simulink library "Generator_Lib"  (R2014a)
settings: Solver=ode45  StartTime=0.0  StopTime=10.0  RelTol=1e-3
undefined symbols (not defined in the file): block_angle, D1, Delta, DiscIntNeverNeededParam, fao, gcbh, sps_rtmsupport, Ts
libraries: powerlib x73, simulink x16, powerlib_extras x13, Generator_Lib x3, sps_avr x2, powerlib_meascontrol x2, spsSimpleSynchronousMachineModel x2
(part 2 of 3)

== system Generator_Lib/Cyclo Gen/Ideal/Phase C Cycloconverter ==
  negative cycle : powerlib/Power Electronics/Universal Bridge  Arms=3  SnubberResistance=1e3  SnubberCapacitance=1e-7  Device=Thyristors  Ron=1e-5  Lon=0  ForwardVoltages="[  0  0  ]"  ForwardVoltage=0  GTOparameters=[ 10e-6 , 20e-6 ]  IGBTparameters=[ 1e-6 , 2e-6 ]  Measurements=None  Measurements_2=None  converterType=Rectifier
  positive cycle : powerlib/Power Electronics/Universal Bridge  Arms=3  SnubberResistance=1e3  SnubberCapacitance=1e-7  Device=Thyristors  Ron=1e-5  Lon=0  ForwardVoltages="[  0  0  ]"  ForwardVoltage=0  GTOparameters=[ 10e-6 , 20e-6 ]  IGBTparameters=[ 1e-6 , 2e-6 ]  Measurements=None  Measurements_2=None  converterType=Rectifier
  VC+ : PMIOPort  Tag=PMCPort  Port=1  Side=Right
  VC- : PMIOPort  Tag=PMCPort  Port=2  Side=Right
  A : PMIOPort  Tag=PMCPort  Port=3  Side=Left
  B : PMIOPort  Tag=PMCPort  Port=4  Side=Left
  C : PMIOPort  Tag=PMCPort  Port=5  Side=Left
  wires:
  [PhCgp] -> positive cycle/1
  [PhCgn] -> negative cycle/1
  connections:
  A/RConn1 -- positive cycle/LConn1 -- negative cycle/LConn1
  B/RConn1 -- positive cycle/LConn2 -- negative cycle/LConn2
  C/RConn1 -- positive cycle/LConn3 -- negative cycle/LConn3
  negative cycle/RConn1 -- positive cycle/RConn2 -- VC-/RConn1
  positive cycle/RConn1 -- VC+/RConn1 -- negative cycle/RConn2

== system Generator_Lib/DC Gen/Ideal/Sensing ==
  Constant : Constant  Value=[1 1]*12000  SampleTime=-1
  Constant1 : Constant  Value=202  SampleTime=-1
  Mux : Mux  Inputs=3
  rpm2pu1 : Gain  Gain=2*pi/60
  tag scope: Gen1Data=global
  wires:
  Constant/1 -> rpm2pu1/1  "Spd"
  Mux/1 -> [Gen1Data]
  rpm2pu1/1 -> Mux/1
  Constant1/1 -> Mux/2
  [Pwr_Gen1_Only] -> Mux/3

== system Generator_Lib/DC Gen/Sync Mach/Displays ==
  w : Inport
  Frequency (Hz) : Display
      settings: Decimation=100  SampleTime=1e-2
  Gain : Gain  Gain=30/pi
  Gain3 : Gain  Gain=1/30
  Rate Transition : RateTransition  OutPortSampleTimeOpt=Inherit  OutPortSampleTime=Ts
  Rate Transition1 : RateTransition  OutPortSampleTimeOpt=Inherit  OutPortSampleTime=Ts
  Speed (RPM) : Display
      settings: Decimation=100  SampleTime=1e-2
  wires:
  w/1 -> Gain/1
  Rate Transition/1 -> Speed (RPM)/1
  Gain3/1 -> Rate Transition1/1
  Gain/1 -> Rate Transition/1, Gain3/1
  Rate Transition1/1 -> Frequency (Hz)/1

== system Generator_Lib/DC Gen/Sync Mach/Generator Control Unit (GCU) ==
  Iabc : Inport
  Vabc : Inport  Port=2
  PMG : Inport  Port=3
  Demux : Demux  Outputs=3
  Excitation System : sps_avr/Excitation System  tr=20e-3  reg=[ 300, 0.001 ]  exc=[ 1, 0 ]  tgr=[ 0, 0 ]  damp=[ 0.001, 0.1 ]  sat=[ 0, 0 ]  lim=[ -2, 2, 0 ]  v0=[1 1*203.1/200]
  Integrator : Integrator
  PU_SI : Gain  Gain=200
  SI_PU : Gain  Gain=1/(200*sqrt(2))
  Terminator1 : Terminator
  Terminator2 : Terminator
  Vref : Constant
  abc to dq0 : powerlib_meascontrol/Transformations/abc to dq0  Alignment=90 degrees behind phase A axis
  threshold3 : Constant  Value=0
  V Field : Outport
  tag scope: Gen1_Vfield=global
  wires:
  Vabc/1 -> SI_PU/1
  PMG/1 -> Integrator/1
  Integrator/1 -> abc to dq0/2
  abc to dq0/1 -> Demux/1
  Demux/1 -> Excitation System/2
  Demux/2 -> Excitation System/3
  SI_PU/1 -> abc to dq0/1
  Excitation System/1 -> PU_SI/1
  PU_SI/1 -> V Field/1, [Gen1_Vfield]
  Vref/1 -> Excitation System/1
  threshold3/1 -> Excitation System/4
  Iabc/1 -> Terminator1/1
  Demux/3 -> Terminator2/1

== system Generator_Lib/DC Gen/Sync Mach/Generator Control Breaker (GCB) ==
  GLC : Inport
  Close switch : Subsystem
  Complex to Real-Imag : ComplexToRealImag  Output=Real
  Complex to Real-Imag1 : ComplexToRealImag  Output=Real
  Contactor : Subsystem
  Memory : Memory
  P.O.R  and CTA : powerlib/Measurements/Three-Phase V-I Measurement  VoltageMeasurement=phase-to-phase  SetLabelV=off  LabelV=Vabc_Gen1  Vpu=off  VpuLL=off  CurrentMeasurement=yes  SetLabelI=off  LabelI=Iabc_Gen1  Ipu=off  Pbase=100e6  Vbase=500e3  OutputType=Complex  PhasorSimulation=off  PSBequivalent=0
  in_a : PMIOPort  Port=1  Side=Left
  in_b : PMIOPort  Port=2  Side=Left
  in_c : PMIOPort  Port=3  Side=Left
  out_a : PMIOPort  Port=4  Side=Right
  out_b : PMIOPort  Port=5  Side=Right
  out_c : PMIOPort  Port=6  Side=Right
  Vabc : Outport
  Iabc : Outport  Port=2
  wires:
  Close switch/1(Out1) -> Contactor/1(com)
  Memory/1 -> Close switch/1(In1)
  Complex to Real-Imag1/1 -> Iabc/1
  Complex to Real-Imag/1 -> Vabc/1
  P.O.R  and CTA/2 -> Complex to Real-Imag1/1
  P.O.R  and CTA/1 -> Complex to Real-Imag/1
  GLC/1 -> Memory/1
  connections:
  Contactor/RConn3 -- out_c/RConn1
  Contactor/RConn1 -- out_a/RConn1
  P.O.R  and CTA/RConn2 -- Contactor/LConn2
  Contactor/LConn3 -- P.O.R  and CTA/RConn3
  P.O.R  and CTA/LConn3 -- in_c/RConn1
  in_b/RConn1 -- P.O.R  and CTA/LConn2
  P.O.R  and CTA/LConn1 -- in_a/RConn1
  Contactor/LConn1 -- P.O.R  and CTA/RConn1
  out_b/RConn1 -- Contactor/RConn2

== system Generator_Lib/DC Gen/Sync Mach/Sensing ==
  In1 : Inport
  Data : Subsystem
  Mux : Mux  Inputs=3
  tag scope: Gen1Data=global
  wires:
  Mux/1 -> [Gen1Data]
  In1/1 -> Data/1(B)
  Data/1(w) -> Mux/1
  Data/2(Vf) -> Mux/2
  Data/3(Pe) -> Mux/3

== system Generator_Lib/DC Gen/Sync Mach/Simplified Synchronous Machine SI Units ==
  mec : Inport
  E : Inport  Port=2
  Electrical model : Subsystem  BlockChoice=Continuous
      settings: AttributesFormatString=%<BlockChoice>  TemplateBlock=spsSimpleSynchronousMachineModel/Electrical model  MemberBlocks=Continuous,Discrete,Phasor
  Measurement list : Subsystem
  Mechanical model : Subsystem  BlockChoice=Continuous w input
      settings: AttributesFormatString=%<BlockChoice>  TemplateBlock=spsSimpleSynchronousMachineModel/Mechanical model  MemberBlocks=Continuous Pm input,Continuous w input,Discrete Pm input,Discrete w input,Phasor Pm input,Phasor w input,Shaft input
  SSM : PMComponent  PhysicalDomain=powersysdomain  LeftPortType=p1  RightPortType=p1  LConnTagsString=__newl0  RConnTagsString=A|B|C  mask(InnerPowersysBlock){}
  A : PMIOPort  Port=1  Side=Right
  B : PMIOPort  Port=2  Side=Right
  C : PMIOPort  Port=3  Side=Right
  m : Outport  InitialOutput=0
  tag scope: LibraryTag=global
  wires:
  Mechanical model/2(wm) -> Electrical model/4(wm)
  Mechanical model/1(theta_e) -> Electrical model/3(theta_e)
  E/1 -> Electrical model/2(e)
  [LibraryTag] -> Electrical model/1(v)
  Electrical model/1(i) -> [LibraryTag]
  Electrical model/2(m) -> Measurement list/1(In1)
  mec/1 -> Mechanical model/1(input)  "Pm or w"
  Electrical model/3(Pe) -> Mechanical model/2(Pe)
  Measurement list/1(Out1) -> m/1
  connections:
  SSM/RConn2 -- B/RConn1
  SSM/RConn1 -- A/RConn1
  SSM/RConn3 -- C/RConn1

== system Generator_Lib/DC Gen/Sync Mach/Vab ==
  Voltage Measurement : powerlib/Measurements/Voltage Measurement  PhasorSimulation=off  OutputType=Magnitude  PSBequivalent=0
  + : PMIOPort  Port=1  Side=Right
  - : PMIOPort  Port=2  Side=Right
  tag scope: Gen1_Vab=global
  wires:
  Voltage Measurement/1 -> [Gen1_Vab]
  connections:
  Voltage Measurement/LConn2 -- -/RConn1
  Voltage Measurement/LConn1 -- +/RConn1

== system Generator_Lib/Integrated Drive/Generator Control Breaker (GCB)/Close switch ==
  In1 : Inport
  Data Type Conversion : DataTypeConversion
  Rad_Rpm : Gain  Gain=30/pi
  Relay : Relay  OnSwitchValue=9000  OffSwitchValue=8900
  Out1 : Outport
  wires:
  In1/1 -> Rad_Rpm/1
  Relay/1 -> Data Type Conversion/1
  Rad_Rpm/1 -> Relay/1
  Data Type Conversion/1 -> Out1/1

== system Generator_Lib/Integrated Drive/Generator Control Breaker (GCB)/Contactor ==
  com : Inport
  Three-Phase Breaker : powerlib/Elements/Three-Phase Breaker  InitialState=open  SwitchA=on  SwitchB=on  SwitchC=on  SwitchTimes="[4/60  10/60]"  External=on  BreakerResistance=0.001  SnubberResistance=1e3  SnubberCapacitance=inf  Measurements=None
  A : PMIOPort  Port=1  Side=Left
  a : PMIOPort  Port=2  Side=Right
  B : PMIOPort  Port=3  Side=Left
  b : PMIOPort  Port=4  Side=Right
  C : PMIOPort  Port=5  Side=Left
  c : PMIOPort  Port=6  Side=Right
  wires:
  com/1 -> Three-Phase Breaker/1
  connections:
  C/RConn1 -- Three-Phase Breaker/LConn3
  B/RConn1 -- Three-Phase Breaker/LConn2
  A/RConn1 -- Three-Phase Breaker/LConn1
  c/RConn1 -- Three-Phase Breaker/RConn3
  Three-Phase Breaker/RConn2 -- b/RConn1
  a/RConn1 -- Three-Phase Breaker/RConn1

== system Generator_Lib/Integrated Drive/Sensing/Data ==
  B : Inport
  Bus Selector : BusSelector  OutputSignals=Rotor speed wm (rad/s),Electrical power Pe (W),Terminal voltage Va (V),Terminal voltage Vb (V),Terminal voltage Vc (V),Stator current is_a (A),Stator current is_b (A),Stator current is_c (A)
  Constant : Constant  Value=12000
  Mux : Mux  Inputs=2
  Mux1 : Mux  Inputs=3
  Mux2 : Mux  Inputs=3
  rpm2pu1 : Gain  Gain=2*pi/60
  w : Outport
  Vf : Outport  Port=2
  Pe : Outport  Port=3
  tag scope: Iabc_Gen1Only=global, Vabc_Gen1Only=global
  wires:
  [Gen1_Vfield] -> Vf/1
  B/1 -> Bus Selector/1
  Bus Selector/2 -> Pe/1  "<Electrical power Pe (W)>"
  Bus Selector/1 -> Mux/1  "<Rotor speed wm (rad/s)>"
  rpm2pu1/1 -> Mux/2
  Constant/1 -> rpm2pu1/1  "Spd"
  Mux/1 -> w/1
  Bus Selector/3 -> Mux1/1  "<Terminal voltage Va (V)>"
  Bus Selector/4 -> Mux1/2  "<Terminal voltage Vb (V)>"
  Bus Selector/5 -> Mux1/3  "<Terminal voltage Vc (V)>"
  Mux1/1 -> [Vabc_Gen1Only]
  Mux2/1 -> [Iabc_Gen1Only]
  Bus Selector/6 -> Mux2/1  "<Stator current is_a (A)>"
  Bus Selector/7 -> Mux2/2  "<Stator current is_b (A)>"
  Bus Selector/8 -> Mux2/3  "<Stator current is_c (A)>"

== system Generator_Lib/VSCF Cycloconverter/AC Generator Cycloconverter/Cycloconverter control (Vsync) ==
  Cyclo Firing Control PhA : Subsystem
  Cyclo Firing Control PhB : Subsystem
  Cyclo Firing Control PhC : Subsystem
  Demux : Demux  Outputs=3
  Discrete-Time Integrator : DiscreteIntegrator  SampleTime=Ts  ICPrevOutput=DiscIntNeverNeededParam  ICPrevScaledInput=DiscIntNeverNeededParam
  Gain1 : Gain  Gain=2*pi
  Gain2 : Gain  Gain=1/(200*sqrt(2/3))
  Gain5 : Gain  Gain=200*sqrt(2/3)
  Sine : Subsystem
  output frequency (Hz) : simulink/Sources/Repeating Sequence  rep_seq_t=[0 10]  rep_seq_y=[1 1]*400
  output voltage (V peak) : simulink/Sources/Repeating Sequence  rep_seq_t=[0 10]  rep_seq_y=[1 1]*200*sqrt(2/3)
  tag scope: Ea=global, vab=global, vbc=global, vca=global
  wires:
  Discrete-Time Integrator/1 -> Sine/2(theta)
  Sine/2(b) -> Cyclo Firing Control PhB/1(Eref)
  Sine/1(a) -> Cyclo Firing Control PhA/1(Eref), Gain5/1
  Sine/3(c) -> Cyclo Firing Control PhC/1(Eref)
  output frequency (Hz)/1 -> Gain1/1
  Gain1/1 -> Discrete-Time Integrator/1
  Gain5/1 -> [Ea]
  output voltage (V peak)/1 -> Gain2/1
  Gain2/1 -> Sine/1(Eref)
  [Vsync] -> Demux/1
  Demux/1 -> [vab]
  Demux/2 -> [vbc]
  Demux/3 -> [vca]
  [input_freq] -> Cyclo Firing Control PhC/2(freq (Hz)), Cyclo Firing Control PhA/2(freq (Hz)), Cyclo Firing Control PhB/2(freq (Hz))

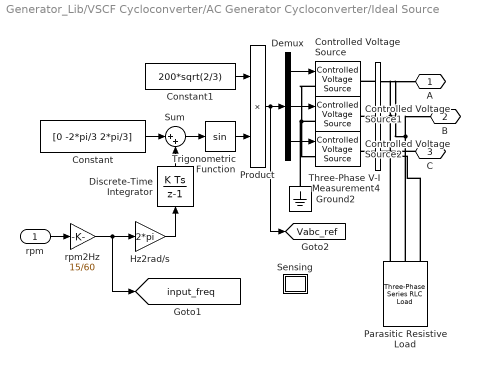
== system Generator_Lib/VSCF Cycloconverter/AC Generator Cycloconverter/Ideal Source ==
  rpm : Inport
  Constant : Constant  Value=[0 -2*pi/3 2*pi/3]
  Constant1 : Constant  Value=200*sqrt(2/3)
  Controlled Voltage Source : powerlib/Electrical Sources/Controlled Voltage Source  Initialize=off  Source_Type=AC  Amplitude=0  Phase=0  Frequency=0  Measurements=None
  Controlled Voltage Source1 : powerlib/Electrical Sources/Controlled Voltage Source  Initialize=off  Source_Type=AC  Amplitude=0  Phase=0  Frequency=0  Measurements=None
  Controlled Voltage Source2 : powerlib/Electrical Sources/Controlled Voltage Source  Initialize=off  Source_Type=AC  Amplitude=0  Phase=0  Frequency=0  Measurements=None
  Demux : Demux  Outputs=3
  Discrete-Time Integrator : DiscreteIntegrator  SampleTime=Ts  ICPrevOutput=DiscIntNeverNeededParam  ICPrevScaledInput=DiscIntNeverNeededParam
  Ground2 : powerlib/Elements/Ground  LConnTagsString=a
  Hz2rad/s : Gain  Gain=2*pi
  Parasitic Resistive Load : powerlib/Elements/Three-Phase Series RLC Load  LConnTagsString=A|B|C  Configuration=Y (grounded)  NominalVoltage=200  NominalFrequency=400  ActivePower=5000  InductivePower=0  CapacitivePower=0  Measurements=None  LoadType=constant Z
  Product : Product
  Sensing : Subsystem
      mask Display: disp('S')
  Sum : Sum  Inputs=|++
  Three-Phase V-I Measurement4 : powerlib/Measurements/Three-Phase V-I Measurement  VoltageMeasurement=phase-to-ground  SetLabelV=on  LabelV=Vabc_Gen1Only  Vpu=off  VpuLL=off  CurrentMeasurement=yes  SetLabelI=on  LabelI=Iabc_Gen1Only  Ipu=off  Pbase=100e6  Vbase=500e3  OutputType=Magnitude  PhasorSimulation=on  PSBequivalent=0
  Trigonometric Function : Trigonometry
  rpm2Hz : Gain  Gain=15/60
  A : PMIOPort  Port=1  Side=Right
  B : PMIOPort  Port=2  Side=Right
  C : PMIOPort  Port=3  Side=Right
  tag scope: Vabc_ref=global, input_freq=global
  wires:
  rpm/1 -> rpm2Hz/1
  Discrete-Time Integrator/1 -> Sum/2
  Constant1/1 -> Product/1
  Constant/1 -> Sum/1
  Hz2rad/s/1 -> Discrete-Time Integrator/1
  Sum/1 -> Trigonometric Function/1
  Trigonometric Function/1 -> Product/2
  Product/1 -> [Vabc_ref], Demux/1
  Demux/1 -> Controlled Voltage Source/1
  Demux/2 -> Controlled Voltage Source1/1
  Demux/3 -> Controlled Voltage Source2/1
  rpm2Hz/1 -> [input_freq], Hz2rad/s/1
  connections:
  Controlled Voltage Source/LConn1 -- Ground2/LConn1 -- Controlled Voltage Source2/LConn1 -- Controlled Voltage Source1/LConn1
  Three-Phase V-I Measurement4/LConn2 -- Controlled Voltage Source1/RConn1
  Three-Phase V-I Measurement4/LConn1 -- Controlled Voltage Source/RConn1
  Three-Phase V-I Measurement4/LConn3 -- Controlled Voltage Source2/RConn1
  C/RConn1 -- Parasitic Resistive Load/LConn3 -- Three-Phase V-I Measurement4/RConn3
  Three-Phase V-I Measurement4/RConn2 -- B/RConn1 -- Parasitic Resistive Load/LConn2
  Three-Phase V-I Measurement4/RConn1 -- A/RConn1 -- Parasitic Resistive Load/LConn1

== system Generator_Lib/VSCF Cycloconverter/AC Generator Cycloconverter/Phase A Cycloconverter ==
  negative cycle : powerlib/Power Electronics/Universal Bridge  Arms=3  SnubberResistance=1e3  SnubberCapacitance=1e-7  Device=Thyristors  Ron=1e-5  Lon=0  ForwardVoltages="[  0  0  ]"  ForwardVoltage=0  GTOparameters=[ 10e-6 , 20e-6 ]  IGBTparameters=[ 1e-6 , 2e-6 ]  Measurements=None  Measurements_2=None  converterType=Rectifier
  positive cycle : powerlib/Power Electronics/Universal Bridge  Arms=3  SnubberResistance=1e3  SnubberCapacitance=1e-7  Device=Thyristors  Ron=1e-5  Lon=0  ForwardVoltages="[  0  0  ]"  ForwardVoltage=0  GTOparameters=[ 10e-6 , 20e-6 ]  IGBTparameters=[ 1e-6 , 2e-6 ]  Measurements=None  Measurements_2=None  converterType=Rectifier
  VA+ : PMIOPort  Tag=PMCPort  Port=1  Side=Right
  VA- : PMIOPort  Tag=PMCPort  Port=2  Side=Right
  A : PMIOPort  Tag=PMCPort  Port=3  Side=Left
  B : PMIOPort  Tag=PMCPort  Port=4  Side=Left
  C : PMIOPort  Tag=PMCPort  Port=5  Side=Left
  wires:
  [PhAgp] -> positive cycle/1
  [PhAgn] -> negative cycle/1
  connections:
  A/RConn1 -- positive cycle/LConn1 -- negative cycle/LConn1
  B/RConn1 -- positive cycle/LConn2 -- negative cycle/LConn2
  C/RConn1 -- positive cycle/LConn3 -- negative cycle/LConn3
  negative cycle/RConn1 -- positive cycle/RConn2 -- VA-/RConn1
  positive cycle/RConn1 -- VA+/RConn1 -- negative cycle/RConn2

== system Generator_Lib/VSCF Cycloconverter/AC Generator Cycloconverter/Phase B Cycloconverter ==
  negative cycle : powerlib/Power Electronics/Universal Bridge  Arms=3  SnubberResistance=1e3  SnubberCapacitance=1e-7  Device=Thyristors  Ron=1e-5  Lon=0  ForwardVoltages="[  0  0  ]"  ForwardVoltage=0  GTOparameters=[ 10e-6 , 20e-6 ]  IGBTparameters=[ 1e-6 , 2e-6 ]  Measurements=None  Measurements_2=None  converterType=Rectifier
  positive cycle : powerlib/Power Electronics/Universal Bridge  Arms=3  SnubberResistance=1e3  SnubberCapacitance=1e-7  Device=Thyristors  Ron=1e-5  Lon=0  ForwardVoltages="[  0  0  ]"  ForwardVoltage=0  GTOparameters=[ 10e-6 , 20e-6 ]  IGBTparameters=[ 1e-6 , 2e-6 ]  Measurements=None  Measurements_2=None  converterType=Rectifier
  VB+ : PMIOPort  Tag=PMCPort  Port=1  Side=Right
  VB- : PMIOPort  Tag=PMCPort  Port=2  Side=Right
  A : PMIOPort  Tag=PMCPort  Port=3  Side=Left
  B : PMIOPort  Tag=PMCPort  Port=4  Side=Left
  C : PMIOPort  Tag=PMCPort  Port=5  Side=Left
  wires:
  [PhBgn] -> negative cycle/1
  [PhBgp] -> positive cycle/1
  connections:
  negative cycle/RConn2 -- VB+/RConn1 -- positive cycle/RConn1
  VB-/RConn1 -- positive cycle/RConn2 -- negative cycle/RConn1
  negative cycle/LConn3 -- positive cycle/LConn3 -- C/RConn1
  negative cycle/LConn2 -- B/RConn1 -- positive cycle/LConn2
  negative cycle/LConn1 -- positive cycle/LConn1 -- A/RConn1

== system Generator_Lib/VSCF Cycloconverter/AC Generator Cycloconverter/Phase C Cycloconverter ==
  negative cycle : powerlib/Power Electronics/Universal Bridge  Arms=3  SnubberResistance=1e3  SnubberCapacitance=1e-7  Device=Thyristors  Ron=1e-5  Lon=0  ForwardVoltages="[  0  0  ]"  ForwardVoltage=0  GTOparameters=[ 10e-6 , 20e-6 ]  IGBTparameters=[ 1e-6 , 2e-6 ]  Measurements=None  Measurements_2=None  converterType=Rectifier
  positive cycle : powerlib/Power Electronics/Universal Bridge  Arms=3  SnubberResistance=1e3  SnubberCapacitance=1e-7  Device=Thyristors  Ron=1e-5  Lon=0  ForwardVoltages="[  0  0  ]"  ForwardVoltage=0  GTOparameters=[ 10e-6 , 20e-6 ]  IGBTparameters=[ 1e-6 , 2e-6 ]  Measurements=None  Measurements_2=None  converterType=Rectifier
  VC+ : PMIOPort  Tag=PMCPort  Port=1  Side=Right
  VC- : PMIOPort  Tag=PMCPort  Port=2  Side=Right
  A : PMIOPort  Tag=PMCPort  Port=3  Side=Left
  B : PMIOPort  Tag=PMCPort  Port=4  Side=Left
  C : PMIOPort  Tag=PMCPort  Port=5  Side=Left
  wires:
  [PhCgp] -> positive cycle/1
  [PhCgn] -> negative cycle/1
  connections:
  A/RConn1 -- positive cycle/LConn1 -- negative cycle/LConn1
  B/RConn1 -- positive cycle/LConn2 -- negative cycle/LConn2
  C/RConn1 -- positive cycle/LConn3 -- negative cycle/LConn3
  negative cycle/RConn1 -- positive cycle/RConn2 -- VC-/RConn1
  positive cycle/RConn1 -- VC+/RConn1 -- negative cycle/RConn2

== system Generator_Lib/VSCF Cycloconverter/Generator Control Breaker (GCB)/Close switch ==
  In1 : Inport
  Data Type Conversion : DataTypeConversion
  Rad_Rpm : Gain  Gain=30/pi
  Relay : Relay  OnSwitchValue=9000  OffSwitchValue=8900
  Out1 : Outport
  wires:
  In1/1 -> Rad_Rpm/1
  Relay/1 -> Data Type Conversion/1
  Rad_Rpm/1 -> Relay/1
  Data Type Conversion/1 -> Out1/1

== system Generator_Lib/VSCF Cycloconverter/Generator Control Breaker (GCB)/Contactor ==
  com : Inport
  Three-Phase Breaker : powerlib/Elements/Three-Phase Breaker  InitialState=open  SwitchA=on  SwitchB=on  SwitchC=on  SwitchTimes="[4/60  10/60]"  External=on  BreakerResistance=0.001  SnubberResistance=1e3  SnubberCapacitance=inf  Measurements=None
  A : PMIOPort  Port=1  Side=Left
  a : PMIOPort  Port=2  Side=Right
  B : PMIOPort  Port=3  Side=Left
  b : PMIOPort  Port=4  Side=Right
  C : PMIOPort  Port=5  Side=Left
  c : PMIOPort  Port=6  Side=Right
  wires:
  com/1 -> Three-Phase Breaker/1
  connections:
  C/RConn1 -- Three-Phase Breaker/LConn3
  B/RConn1 -- Three-Phase Breaker/LConn2
  A/RConn1 -- Three-Phase Breaker/LConn1
  c/RConn1 -- Three-Phase Breaker/RConn3
  Three-Phase Breaker/RConn2 -- b/RConn1
  a/RConn1 -- Three-Phase Breaker/RConn1

== system Generator_Lib/VSCF DC Link/Rect and Inv/Subsystem3 ==
  Vdc : powerlib/Measurements/Voltage Measurement  Tag=PoWeRsYsTeMmEaSuReMeNt  PhasorSimulation=off  OutputType=Magnitude  PSBequivalent=0
  + : PMIOPort  Port=1  Side=Left
  - : PMIOPort  Port=2  Side=Right
  tag scope: Vdc_GenDCLink=global
  wires:
  Vdc/1 -> [Vdc_GenDCLink]  "Vdc"
  connections:
  Vdc/LConn1 -- +/RConn1
  -/RConn1 -- Vdc/LConn2

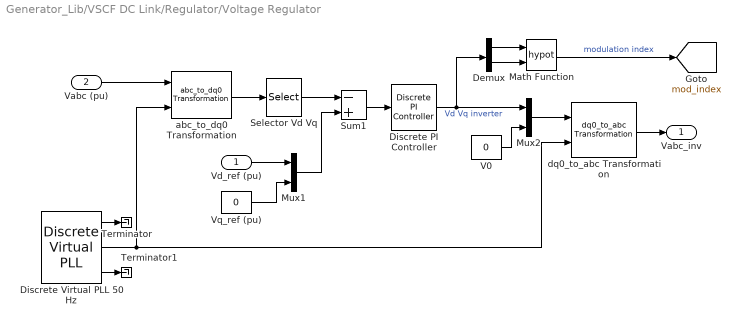
== system Generator_Lib/VSCF DC Link/Regulator/Voltage Regulator ==
  Vd_ref (pu) : Inport
  Vabc (pu) : Inport  Port=2
  Demux : Demux  Outputs=2
  Discrete PI Controller : powerlib_extras/Discrete  Control Blocks/Discrete PI Controller  Kp=Kp  Ki=Ki  Par_Limits=[1 -1]  Init=0  Ts=Ts
  Discrete Virtual PLL 50 Hz : powerlib_extras/Discrete  Control Blocks/Discrete Virtual PLL  Freq=400  Phase=0  Ts=Ts
  Math Function : Math  Operator=hypot  SaturateOnIntegerOverflow=on
  Mux1 : Mux  Inputs=2
  Mux2 : Mux  Inputs=2
  Selector Vd Vq : Selector  InputPortWidth=3  Indices=[1 2]
  Sum1 : Sum  Inputs=-+  SaturateOnIntegerOverflow=on  InputSameDT=on  OutDataTypeStr=Inherit: Same as first input
  Terminator : Terminator
  Terminator1 : Terminator
  V0 : Constant  Value=0
  Vq_ref (pu) : Constant  Value=0
  abc_to_dq0 Transformation : powerlib_extras/Measurements/abc_to_dq0 Transformation
  dq0_to_abc Transformation : powerlib_extras/Measurements/dq0_to_abc Transformation
  Vabc_inv : Outport
  tag scope: mod_index=global
  wires:
  abc_to_dq0 Transformation/1 -> Selector Vd Vq/1
  Vabc (pu)/1 -> abc_to_dq0 Transformation/1
  Selector Vd Vq/1 -> Sum1/1
  Sum1/1 -> Discrete PI Controller/1
  Mux2/1 -> dq0_to_abc Transformation/1
  V0/1 -> Mux2/2
  dq0_to_abc Transformation/1 -> Vabc_inv/1
  Discrete Virtual PLL 50 Hz/2 -> abc_to_dq0 Transformation/2, dq0_to_abc Transformation/2
  Vd_ref (pu)/1 -> Mux1/1
  Vq_ref (pu)/1 -> Mux1/2
  Mux1/1 -> Sum1/2
  Discrete Virtual PLL 50 Hz/1 -> Terminator/1
  Discrete Virtual PLL 50 Hz/3 -> Terminator1/1
  Discrete PI Controller/1 -> Demux/1, Mux2/1  "Vd Vq inverter"
  Demux/1 -> Math Function/1
  Demux/2 -> Math Function/2
  Math Function/1 -> [mod_index]  "modulation index"

== system Generator_Lib/Cyclo Gen/Ideal/Cycloconverter control (Vsync)/Cyclo Firing Control PhA ==
  Eref : Inport
  freq (Hz) : Inport  Port=2
  Compare To Constant : simulink/Logic and Bit Operations/Compare To Constant  relop=>=  const=block_angle  OutDataTypeStr=boolean  ZeroCross=off
  Compare To Constant1 : simulink/Logic and Bit Operations/Compare To Constant  relop=>  const=block_angle  OutDataTypeStr=boolean  ZeroCross=off
  Discrete Synchronized 6-Pulse Generator (negative) : powerlib_extras/Discrete  Control Blocks/Discrete Synchronized 6-Pulse Generator  pwidth=150  Double_Pulse=off  Ts=Ts
  Discrete Synchronized 6-Pulse Generator (positive) : powerlib_extras/Discrete  Control Blocks/Discrete Synchronized 6-Pulse Generator  pwidth=150  Double_Pulse=off  Ts=Ts
  Gain2 : Gain  Gain=-1
  Lookup Table (negative) : Lookup  InputValues=[-1 0 1]  Table=[90 90 0]+fao
  Lookup Table (positive) : Lookup  InputValues=[-1 0 1]  Table=[90 90 0]+fao
  tag scope: PhAgn=global, PhAgp=global
  wires:
  Discrete Synchronized 6-Pulse Generator (positive)/1 -> [PhAgp]
  Discrete Synchronized 6-Pulse Generator (negative)/1 -> [PhAgn]
  [vca] -> Discrete Synchronized 6-Pulse Generator (positive)/4
  [vbc] -> Discrete Synchronized 6-Pulse Generator (positive)/3
  [vab] -> Discrete Synchronized 6-Pulse Generator (positive)/2
  [vab] -> Discrete Synchronized 6-Pulse Generator (negative)/2
  [vbc] -> Discrete Synchronized 6-Pulse Generator (negative)/3
  [vca] -> Discrete Synchronized 6-Pulse Generator (negative)/4
  Compare To Constant/1 -> Discrete Synchronized 6-Pulse Generator (positive)/6
  Lookup Table (positive)/1 -> Compare To Constant/1, Discrete Synchronized 6-Pulse Generator (positive)/1  "alpha_pos"
  Lookup Table (negative)/1 -> Discrete Synchronized 6-Pulse Generator (negative)/1, Compare To Constant1/1  "alpa_neg"
  Eref/1 -> Lookup Table (positive)/1, Gain2/1
  Compare To Constant1/1 -> Discrete Synchronized 6-Pulse Generator (negative)/6
  Gain2/1 -> Lookup Table (negative)/1
  freq (Hz)/1 -> Discrete Synchronized 6-Pulse Generator (positive)/5, Discrete Synchronized 6-Pulse Generator (negative)/5

== system Generator_Lib/Cyclo Gen/Ideal/Cycloconverter control (Vsync)/Cyclo Firing Control PhB ==
  Eref : Inport
  freq (Hz) : Inport  Port=2
  Compare To Constant : simulink/Logic and Bit Operations/Compare To Constant  relop=>=  const=block_angle  OutDataTypeStr=boolean  ZeroCross=off
  Compare To Constant1 : simulink/Logic and Bit Operations/Compare To Constant  relop=>  const=block_angle  OutDataTypeStr=boolean  ZeroCross=off
  Discrete Synchronized 6-Pulse Generator : powerlib_extras/Discrete  Control Blocks/Discrete Synchronized 6-Pulse Generator  pwidth=150  Double_Pulse=off  Ts=Ts
  Discrete Synchronized 6-Pulse Generator1 : Subsystem  DialogController=POWERSYS.PowerSysDialog  mask(Discrete Synchronized 6-pulse generator){pwidth=150, Double_Pulse=off, Ts=Ts}
      mask prompts: pwidth "Pulse width (degrees) :"; Double_Pulse "Double pulsing"; Ts "Time step (s) :"
      mask help:
      | Use this block to fire the 6 thyristors of a 6-pulse converter.
      |
      | The output is a vector of 6 pulses (0-1) individually synchronized on the 6 commutation voltages. Pulses are generated alpha degrees after the increasing zero-crossings of the commutation voltages.
      |
      | Input 1 is  the alpha firing signal (degrees).
      | Inputs 2, 3 and 4 are the synchronization voltages AB BC CA which should be in phase with the 3 phase-phase voltages at the converter terminals.
      | Input 5: Frequency of the synchronization voltages (use a constant or the Freq PLL output)
      | Input 6 allows  blocking of the pulses when the applied signal is non zero.
      |
      | When the 'Douple pulsing' option is checked, two pulses are sent to each thyristor: a 1st pulse when the aplha angle is reached, then a 2nd pulse 60 degrees later, when the next thyristor is fired.
      mask init:
      | power_initmask();
      mask Help: This block is part of a subset of blocks in the Extras library that does not have documentation associated with it, other than the block mask description.
      mask Display: plot(0,0,100,100,[80 62 62 47 47 30],[40 40 60 60 40 40]-5)
  Gain2 : Gain  Gain=-1
  Lookup Table : Lookup  InputValues=[-1 0 1]  Table=[90 90 0]+fao
  Lookup Table1 : Lookup  InputValues=[-1 0 1]  Table=[90 90 0]+fao
  tag scope: PhBgn=global, PhBgp=global
  wires:
  Eref/1 -> Lookup Table/1, Gain2/1
  Lookup Table1/1 -> Compare To Constant1/1, Discrete Synchronized 6-Pulse Generator1/1(alpha_deg)  "alpa_neg_B"
  Lookup Table/1 -> Compare To Constant/1, Discrete Synchronized 6-Pulse Generator/1  "alpha_pos_B"
  Compare To Constant/1 -> Discrete Synchronized 6-Pulse Generator/6
  [vca] -> Discrete Synchronized 6-Pulse Generator1/4(CA)
  [vbc] -> Discrete Synchronized 6-Pulse Generator1/3(BC)
  [vab] -> Discrete Synchronized 6-Pulse Generator1/2(AB)
  [vab] -> Discrete Synchronized 6-Pulse Generator/2
  [vbc] -> Discrete Synchronized 6-Pulse Generator/3
  [vca] -> Discrete Synchronized 6-Pulse Generator/4
  Discrete Synchronized 6-Pulse Generator1/1(pulses) -> [PhBgn]
  Discrete Synchronized 6-Pulse Generator/1 -> [PhBgp]
  Compare To Constant1/1 -> Discrete Synchronized 6-Pulse Generator1/6(Block)
  Gain2/1 -> Lookup Table1/1
  freq (Hz)/1 -> Discrete Synchronized 6-Pulse Generator1/5(Freq), Discrete Synchronized 6-Pulse Generator/5

== system Generator_Lib/Cyclo Gen/Ideal/Cycloconverter control (Vsync)/Cyclo Firing Control PhC ==
  Eref : Inport
  freq (Hz) : Inport  Port=2
  Compare To Constant : simulink/Logic and Bit Operations/Compare To Constant  relop=>=  const=block_angle  OutDataTypeStr=boolean  ZeroCross=off
  Compare To Constant1 : simulink/Logic and Bit Operations/Compare To Constant  relop=>  const=block_angle  OutDataTypeStr=boolean  ZeroCross=off
  Discrete Synchronized 6-Pulse Generator : powerlib_extras/Discrete  Control Blocks/Discrete Synchronized 6-Pulse Generator  pwidth=120  Double_Pulse=off  Ts=Ts
  Discrete Synchronized 6-Pulse Generator1 : Subsystem  DialogController=POWERSYS.PowerSysDialog  mask(Discrete Synchronized 6-pulse generator){pwidth=120, Double_Pulse=off, Ts=Ts}
      mask prompts: pwidth "Pulse width (degrees) :"; Double_Pulse "Double pulsing"; Ts "Time step (s) :"
      mask help:
      | Use this block to fire the 6 thyristors of a 6-pulse converter.
      |
      | The output is a vector of 6 pulses (0-1) individually synchronized on the 6 commutation voltages. Pulses are generated alpha degrees after the increasing zero-crossings of the commutation voltages.
      |
      | Input 1 is  the alpha firing signal (degrees).
      | Inputs 2, 3 and 4 are the synchronization voltages AB BC CA which should be in phase with the 3 phase-phase voltages at the converter terminals.
      | Input 5: Frequency of the synchronization voltages (use a constant or the Freq PLL output)
      | Input 6 allows  blocking of the pulses when the applied signal is non zero.
      |
      | When the 'Douple pulsing' option is checked, two pulses are sent to each thyristor: a 1st pulse when the aplha angle is reached, then a 2nd pulse 60 degrees later, when the next thyristor is fired.
      mask init:
      | power_initmask();
      mask Help: This block is part of a subset of blocks in the Extras library that does not have documentation associated with it, other than the block mask description.
      mask Display: plot(0,0,100,100,[80 62 62 47 47 30],[40 40 60 60 40 40]-5)
  Gain2 : Gain  Gain=-1
  Lookup Table : Lookup  InputValues=[-1 0 1]  Table=[90 90 0]+fao
  Lookup Table1 : Lookup  InputValues=[-1 0 1]  Table=[90 90 0]+fao
  tag scope: PhCgn=global, PhCgp=global
  wires:
  Discrete Synchronized 6-Pulse Generator/1 -> [PhCgp]
  Discrete Synchronized 6-Pulse Generator1/1(pulses) -> [PhCgn]
  [vca] -> Discrete Synchronized 6-Pulse Generator/4
  [vbc] -> Discrete Synchronized 6-Pulse Generator/3
  [vab] -> Discrete Synchronized 6-Pulse Generator/2
  [vab] -> Discrete Synchronized 6-Pulse Generator1/2(AB)
  [vbc] -> Discrete Synchronized 6-Pulse Generator1/3(BC)
  [vca] -> Discrete Synchronized 6-Pulse Generator1/4(CA)
  Compare To Constant/1 -> Discrete Synchronized 6-Pulse Generator/6
  Lookup Table/1 -> Compare To Constant/1, Discrete Synchronized 6-Pulse Generator/1  "alpha_pos_C"
  Lookup Table1/1 -> Compare To Constant1/1, Discrete Synchronized 6-Pulse Generator1/1(alpha_deg)  "alpa_neg_C"
  Eref/1 -> Lookup Table/1, Gain2/1
  Compare To Constant1/1 -> Discrete Synchronized 6-Pulse Generator1/6(Block)
  freq (Hz)/1 -> Discrete Synchronized 6-Pulse Generator1/5(Freq), Discrete Synchronized 6-Pulse Generator/5
  Gain2/1 -> Lookup Table1/1

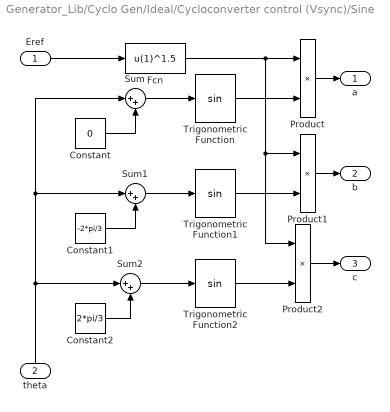
== system Generator_Lib/Cyclo Gen/Ideal/Cycloconverter control (Vsync)/Sine ==
  Eref : Inport
  theta : Inport  Port=2
  Constant : Constant  Value=0
  Constant1 : Constant  Value=-2*pi/3
  Constant2 : Constant  Value=2*pi/3
  Fcn : Fcn  Expr=u(1)^1.5
  Product : Product  RndMeth=Zero
  Product1 : Product  RndMeth=Zero
  Product2 : Product  RndMeth=Zero
  Sum : Sum  Inputs=|++
  Sum1 : Sum  Inputs=|++
  Sum2 : Sum  Inputs=|++
  Trigonometric Function : Trigonometry
  Trigonometric Function1 : Trigonometry
  Trigonometric Function2 : Trigonometry
  a : Outport
  b : Outport  Port=2
  c : Outport  Port=3
  wires:
  theta/1 -> Sum1/1, Sum/1, Sum2/1
  Sum/1 -> Trigonometric Function/1
  Constant/1 -> Sum/2
  Trigonometric Function/1 -> Product/2
  Sum1/1 -> Trigonometric Function1/1
  Constant1/1 -> Sum1/2
  Trigonometric Function1/1 -> Product1/2
  Sum2/1 -> Trigonometric Function2/1
  Constant2/1 -> Sum2/2
  Trigonometric Function2/1 -> Product2/2
  Product/1 -> a/1
  Product1/1 -> b/1
  Product2/1 -> c/1
  Eref/1 -> Fcn/1
  Fcn/1 -> Product/1, Product1/1, Product2/1

== system Generator_Lib/Cyclo Gen/Ideal/Ideal Source/Sensing ==
  Constant : Constant  Value=[1 1]*12000  SampleTime=-1
  Constant1 : Constant  Value=202  SampleTime=-1
  Mux : Mux  Inputs=3
  rpm2pu1 : Gain  Gain=2*pi/60
  tag scope: Gen1Data=global
  wires:
  [Pwr_Gen1_Only] -> Mux/3
  Constant1/1 -> Mux/2
  rpm2pu1/1 -> Mux/1
  Mux/1 -> [Gen1Data]
  Constant/1 -> rpm2pu1/1  "Spd"

== system Generator_Lib/DC Gen/Sync Mach/Generator Control Breaker (GCB)/Close switch ==
  In1 : Inport
  Data Type Conversion : DataTypeConversion
  Rad_Rpm : Gain  Gain=30/pi
  Relay : Relay  OnSwitchValue=9000  OffSwitchValue=8900
  Out1 : Outport
  wires:
  In1/1 -> Rad_Rpm/1
  Relay/1 -> Data Type Conversion/1
  Rad_Rpm/1 -> Relay/1
  Data Type Conversion/1 -> Out1/1

== system Generator_Lib/DC Gen/Sync Mach/Generator Control Breaker (GCB)/Contactor ==
  com : Inport
  Three-Phase Breaker : powerlib/Elements/Three-Phase Breaker  InitialState=open  SwitchA=on  SwitchB=on  SwitchC=on  SwitchTimes="[4/60  10/60]"  External=on  BreakerResistance=0.001  SnubberResistance=1e3  SnubberCapacitance=inf  Measurements=None
  A : PMIOPort  Port=1  Side=Left
  a : PMIOPort  Port=2  Side=Right
  B : PMIOPort  Port=3  Side=Left
  b : PMIOPort  Port=4  Side=Right
  C : PMIOPort  Port=5  Side=Left
  c : PMIOPort  Port=6  Side=Right
  wires:
  com/1 -> Three-Phase Breaker/1
  connections:
  C/RConn1 -- Three-Phase Breaker/LConn3
  B/RConn1 -- Three-Phase Breaker/LConn2
  A/RConn1 -- Three-Phase Breaker/LConn1
  c/RConn1 -- Three-Phase Breaker/RConn3
  Three-Phase Breaker/RConn2 -- b/RConn1
  a/RConn1 -- Three-Phase Breaker/RConn1

== system Generator_Lib/DC Gen/Sync Mach/Sensing/Data ==
  B : Inport
  Bus Selector : BusSelector  OutputSignals=Rotor speed wm (rad/s),Electrical power Pe (W),Terminal voltage Va (V),Terminal voltage Vb (V),Terminal voltage Vc (V),Stator current is_a (A),Stator current is_b (A),Stator current is_c (A)
  Constant : Constant  Value=12000
  Mux : Mux  Inputs=2
  Mux1 : Mux  Inputs=3
  Mux2 : Mux  Inputs=3
  rpm2pu1 : Gain  Gain=2*pi/60
  w : Outport
  Vf : Outport  Port=2
  Pe : Outport  Port=3
  tag scope: Iabc_Gen1Only=global, Vabc_Gen1Only=global
  wires:
  [Gen1_Vfield] -> Vf/1
  B/1 -> Bus Selector/1
  Bus Selector/2 -> Pe/1  "<Electrical power Pe (W)>"
  Bus Selector/1 -> Mux/1  "<Rotor speed wm (rad/s)>"
  rpm2pu1/1 -> Mux/2
  Constant/1 -> rpm2pu1/1  "Spd"
  Mux/1 -> w/1
  Bus Selector/3 -> Mux1/1  "<Terminal voltage Va (V)>"
  Bus Selector/4 -> Mux1/2  "<Terminal voltage Vb (V)>"
  Bus Selector/5 -> Mux1/3  "<Terminal voltage Vc (V)>"
  Mux1/1 -> [Vabc_Gen1Only]
  Mux2/1 -> [Iabc_Gen1Only]
  Bus Selector/6 -> Mux2/1  "<Stator current is_a (A)>"
  Bus Selector/7 -> Mux2/2  "<Stator current is_b (A)>"
  Bus Selector/8 -> Mux2/3  "<Stator current is_c (A)>"

== system Generator_Lib/DC Gen/Sync Mach/Simplified Synchronous Machine SI Units/Electrical model ==
  v : Inport
  e : Inport  Port=2
  theta_e : Inport  Port=3
  wm : Inport  Port=4
  Continuous : spsSimpleSynchronousMachineModel/Continuous
  i : Outport
  m : Outport  Port=2
  Pe : Outport  Port=3
  wires:
  v/1 -> Continuous/1
  e/1 -> Continuous/2
  theta_e/1 -> Continuous/3
  wm/1 -> Continuous/4
  Continuous/1 -> i/1
  Continuous/2 -> m/1
  Continuous/3 -> Pe/1

== system Generator_Lib/DC Gen/Sync Mach/Simplified Synchronous Machine SI Units/Measurement list ==
  In1 : Inport
  Bus Creator1 : BusCreator  Inputs=12
  Demux : Demux  Outputs=[1,1,1,1,1,1,1,1,1,1,1,1]
  Out1 : Outport
  wires:
  Demux/12 -> Bus Creator1/12  "Electrical power Pe (W)"
  Demux/11 -> Bus Creator1/11  "Rotor speed wm (rad/s)"
  Demux/10 -> Bus Creator1/10  "Rotor angle theta (rad)"
  Demux/9 -> Bus Creator1/9  "Internal voltage Ec (V)"
  Demux/8 -> Bus Creator1/8  "Internal voltage Eb (V)"
  Demux/7 -> Bus Creator1/7  "Internal voltage Ea (V)"
  Demux/6 -> Bus Creator1/6  "Terminal voltage Vc (V)"
  Demux/5 -> Bus Creator1/5  "Terminal voltage Vb (V)"
  Demux/4 -> Bus Creator1/4  "Terminal voltage Va (V)"
  Demux/3 -> Bus Creator1/3  "Stator current is_c (A)"
  Demux/2 -> Bus Creator1/2  "Stator current is_b (A)"
  Demux/1 -> Bus Creator1/1  "Stator current is_a (A)"
  Bus Creator1/1 -> Out1/1
  In1/1 -> Demux/1

== system Generator_Lib/DC Gen/Sync Mach/Simplified Synchronous Machine SI Units/Mechanical model ==
  input : Inport
  Pe : Inport  Port=2
  Continuous w input : spsSimpleSynchronousMachineModel/Continuous w input
  Shaft : PMIOPort  Port=1  Side=Left
  theta_e : Outport
  wm : Outport  Port=2
  wires:
  input/1 -> Continuous w input/1
  Pe/1 -> Continuous w input/2
  Continuous w input/1 -> theta_e/1
  Continuous w input/2 -> wm/1

== system Generator_Lib/VSCF Cycloconverter/AC Generator Cycloconverter/Cycloconverter control (Vsync)/Cyclo Firing Control PhA ==
  Eref : Inport
  freq (Hz) : Inport  Port=2
  Compare To Constant : simulink/Logic and Bit Operations/Compare To Constant  relop=>=  const=block_angle  OutDataTypeStr=boolean  ZeroCross=off
  Compare To Constant1 : simulink/Logic and Bit Operations/Compare To Constant  relop=>  const=block_angle  OutDataTypeStr=boolean  ZeroCross=off
  Discrete Synchronized 6-Pulse Generator (negative) : powerlib_extras/Discrete  Control Blocks/Discrete Synchronized 6-Pulse Generator  pwidth=150  Double_Pulse=off  Ts=Ts
  Discrete Synchronized 6-Pulse Generator (positive) : powerlib_extras/Discrete  Control Blocks/Discrete Synchronized 6-Pulse Generator  pwidth=150  Double_Pulse=off  Ts=Ts
  Gain2 : Gain  Gain=-1
  Lookup Table (negative) : Lookup  InputValues=[-1 0 1]  Table=[90 90 0]+fao
  Lookup Table (positive) : Lookup  InputValues=[-1 0 1]  Table=[90 90 0]+fao
  tag scope: PhAgn=global, PhAgp=global
  wires:
  Discrete Synchronized 6-Pulse Generator (positive)/1 -> [PhAgp]
  Discrete Synchronized 6-Pulse Generator (negative)/1 -> [PhAgn]
  [vca] -> Discrete Synchronized 6-Pulse Generator (positive)/4
  [vbc] -> Discrete Synchronized 6-Pulse Generator (positive)/3
  [vab] -> Discrete Synchronized 6-Pulse Generator (positive)/2
  [vab] -> Discrete Synchronized 6-Pulse Generator (negative)/2
  [vbc] -> Discrete Synchronized 6-Pulse Generator (negative)/3
  [vca] -> Discrete Synchronized 6-Pulse Generator (negative)/4
  Compare To Constant/1 -> Discrete Synchronized 6-Pulse Generator (positive)/6
  Lookup Table (positive)/1 -> Compare To Constant/1, Discrete Synchronized 6-Pulse Generator (positive)/1  "alpha_pos"
  Lookup Table (negative)/1 -> Discrete Synchronized 6-Pulse Generator (negative)/1, Compare To Constant1/1  "alpa_neg"
  Eref/1 -> Lookup Table (positive)/1, Gain2/1
  Compare To Constant1/1 -> Discrete Synchronized 6-Pulse Generator (negative)/6
  Gain2/1 -> Lookup Table (negative)/1
  freq (Hz)/1 -> Discrete Synchronized 6-Pulse Generator (positive)/5, Discrete Synchronized 6-Pulse Generator (negative)/5

== system Generator_Lib/VSCF Cycloconverter/AC Generator Cycloconverter/Cycloconverter control (Vsync)/Cyclo Firing Control PhB ==
  Eref : Inport
  freq (Hz) : Inport  Port=2
  Compare To Constant : simulink/Logic and Bit Operations/Compare To Constant  relop=>=  const=block_angle  OutDataTypeStr=boolean  ZeroCross=off
  Compare To Constant1 : simulink/Logic and Bit Operations/Compare To Constant  relop=>  const=block_angle  OutDataTypeStr=boolean  ZeroCross=off
  Discrete Synchronized 6-Pulse Generator : powerlib_extras/Discrete  Control Blocks/Discrete Synchronized 6-Pulse Generator  pwidth=150  Double_Pulse=off  Ts=Ts
  Discrete Synchronized 6-Pulse Generator1 : Subsystem  DialogController=POWERSYS.PowerSysDialog  mask(Discrete Synchronized 6-pulse generator){pwidth=150, Double_Pulse=off, Ts=Ts}
      mask prompts: pwidth "Pulse width (degrees) :"; Double_Pulse "Double pulsing"; Ts "Time step (s) :"
      mask help:
      | Use this block to fire the 6 thyristors of a 6-pulse converter.
      |
      | The output is a vector of 6 pulses (0-1) individually synchronized on the 6 commutation voltages. Pulses are generated alpha degrees after the increasing zero-crossings of the commutation voltages.
      |
      | Input 1 is  the alpha firing signal (degrees).
      | Inputs 2, 3 and 4 are the synchronization voltages AB BC CA which should be in phase with the 3 phase-phase voltages at the converter terminals.
      | Input 5: Frequency of the synchronization voltages (use a constant or the Freq PLL output)
      | Input 6 allows  blocking of the pulses when the applied signal is non zero.
      |
      | When the 'Douple pulsing' option is checked, two pulses are sent to each thyristor: a 1st pulse when the aplha angle is reached, then a 2nd pulse 60 degrees later, when the next thyristor is fired.
      mask init:
      | power_initmask();
      mask Help: This block is part of a subset of blocks in the Extras library that does not have documentation associated with it, other than the block mask description.
      mask Display: plot(0,0,100,100,[80 62 62 47 47 30],[40 40 60 60 40 40]-5)
  Gain2 : Gain  Gain=-1
  Lookup Table : Lookup  InputValues=[-1 0 1]  Table=[90 90 0]+fao
  Lookup Table1 : Lookup  InputValues=[-1 0 1]  Table=[90 90 0]+fao
  tag scope: PhBgn=global, PhBgp=global
  wires:
  Eref/1 -> Lookup Table/1, Gain2/1
  Lookup Table1/1 -> Compare To Constant1/1, Discrete Synchronized 6-Pulse Generator1/1(alpha_deg)  "alpa_neg_B"
  Lookup Table/1 -> Compare To Constant/1, Discrete Synchronized 6-Pulse Generator/1  "alpha_pos_B"
  Compare To Constant/1 -> Discrete Synchronized 6-Pulse Generator/6
  [vca] -> Discrete Synchronized 6-Pulse Generator1/4(CA)
  [vbc] -> Discrete Synchronized 6-Pulse Generator1/3(BC)
  [vab] -> Discrete Synchronized 6-Pulse Generator1/2(AB)
  [vab] -> Discrete Synchronized 6-Pulse Generator/2
  [vbc] -> Discrete Synchronized 6-Pulse Generator/3
  [vca] -> Discrete Synchronized 6-Pulse Generator/4
  Discrete Synchronized 6-Pulse Generator1/1(pulses) -> [PhBgn]
  Discrete Synchronized 6-Pulse Generator/1 -> [PhBgp]
  Compare To Constant1/1 -> Discrete Synchronized 6-Pulse Generator1/6(Block)
  Gain2/1 -> Lookup Table1/1
  freq (Hz)/1 -> Discrete Synchronized 6-Pulse Generator1/5(Freq), Discrete Synchronized 6-Pulse Generator/5

== system Generator_Lib/VSCF Cycloconverter/AC Generator Cycloconverter/Cycloconverter control (Vsync)/Cyclo Firing Control PhC ==
  Eref : Inport
  freq (Hz) : Inport  Port=2
  Compare To Constant : simulink/Logic and Bit Operations/Compare To Constant  relop=>=  const=block_angle  OutDataTypeStr=boolean  ZeroCross=off
  Compare To Constant1 : simulink/Logic and Bit Operations/Compare To Constant  relop=>  const=block_angle  OutDataTypeStr=boolean  ZeroCross=off
  Discrete Synchronized 6-Pulse Generator : powerlib_extras/Discrete  Control Blocks/Discrete Synchronized 6-Pulse Generator  pwidth=120  Double_Pulse=off  Ts=Ts
  Discrete Synchronized 6-Pulse Generator1 : Subsystem  DialogController=POWERSYS.PowerSysDialog  mask(Discrete Synchronized 6-pulse generator){pwidth=120, Double_Pulse=off, Ts=Ts}
      mask prompts: pwidth "Pulse width (degrees) :"; Double_Pulse "Double pulsing"; Ts "Time step (s) :"
      mask help:
      | Use this block to fire the 6 thyristors of a 6-pulse converter.
      |
      | The output is a vector of 6 pulses (0-1) individually synchronized on the 6 commutation voltages. Pulses are generated alpha degrees after the increasing zero-crossings of the commutation voltages.
      |
      | Input 1 is  the alpha firing signal (degrees).
      | Inputs 2, 3 and 4 are the synchronization voltages AB BC CA which should be in phase with the 3 phase-phase voltages at the converter terminals.
      | Input 5: Frequency of the synchronization voltages (use a constant or the Freq PLL output)
      | Input 6 allows  blocking of the pulses when the applied signal is non zero.
      |
      | When the 'Douple pulsing' option is checked, two pulses are sent to each thyristor: a 1st pulse when the aplha angle is reached, then a 2nd pulse 60 degrees later, when the next thyristor is fired.
      mask init:
      | power_initmask();
      mask Help: This block is part of a subset of blocks in the Extras library that does not have documentation associated with it, other than the block mask description.
      mask Display: plot(0,0,100,100,[80 62 62 47 47 30],[40 40 60 60 40 40]-5)
  Gain2 : Gain  Gain=-1
  Lookup Table : Lookup  InputValues=[-1 0 1]  Table=[90 90 0]+fao
  Lookup Table1 : Lookup  InputValues=[-1 0 1]  Table=[90 90 0]+fao
  tag scope: PhCgn=global, PhCgp=global
  wires:
  Discrete Synchronized 6-Pulse Generator/1 -> [PhCgp]
  Discrete Synchronized 6-Pulse Generator1/1(pulses) -> [PhCgn]
  [vca] -> Discrete Synchronized 6-Pulse Generator/4
  [vbc] -> Discrete Synchronized 6-Pulse Generator/3
  [vab] -> Discrete Synchronized 6-Pulse Generator/2
  [vab] -> Discrete Synchronized 6-Pulse Generator1/2(AB)
  [vbc] -> Discrete Synchronized 6-Pulse Generator1/3(BC)
  [vca] -> Discrete Synchronized 6-Pulse Generator1/4(CA)
  Compare To Constant/1 -> Discrete Synchronized 6-Pulse Generator/6
  Lookup Table/1 -> Compare To Constant/1, Discrete Synchronized 6-Pulse Generator/1  "alpha_pos_C"
  Lookup Table1/1 -> Compare To Constant1/1, Discrete Synchronized 6-Pulse Generator1/1(alpha_deg)  "alpa_neg_C"
  Eref/1 -> Lookup Table/1, Gain2/1
  Compare To Constant1/1 -> Discrete Synchronized 6-Pulse Generator1/6(Block)
  freq (Hz)/1 -> Discrete Synchronized 6-Pulse Generator1/5(Freq), Discrete Synchronized 6-Pulse Generator/5
  Gain2/1 -> Lookup Table1/1

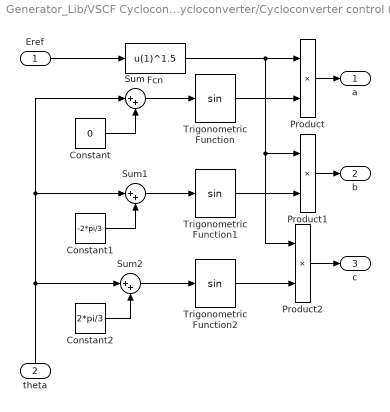
== system Generator_Lib/VSCF Cycloconverter/AC Generator Cycloconverter/Cycloconverter control (Vsync)/Sine ==
  Eref : Inport
  theta : Inport  Port=2
  Constant : Constant  Value=0
  Constant1 : Constant  Value=-2*pi/3
  Constant2 : Constant  Value=2*pi/3
  Fcn : Fcn  Expr=u(1)^1.5
  Product : Product  RndMeth=Zero
  Product1 : Product  RndMeth=Zero
  Product2 : Product  RndMeth=Zero
  Sum : Sum  Inputs=|++
  Sum1 : Sum  Inputs=|++
  Sum2 : Sum  Inputs=|++
  Trigonometric Function : Trigonometry
  Trigonometric Function1 : Trigonometry
  Trigonometric Function2 : Trigonometry
  a : Outport
  b : Outport  Port=2
  c : Outport  Port=3
  wires:
  theta/1 -> Sum1/1, Sum/1, Sum2/1
  Sum/1 -> Trigonometric Function/1
  Constant/1 -> Sum/2
  Trigonometric Function/1 -> Product/2
  Sum1/1 -> Trigonometric Function1/1
  Constant1/1 -> Sum1/2
  Trigonometric Function1/1 -> Product1/2
  Sum2/1 -> Trigonometric Function2/1
  Constant2/1 -> Sum2/2
  Trigonometric Function2/1 -> Product2/2
  Product/1 -> a/1
  Product1/1 -> b/1
  Product2/1 -> c/1
  Eref/1 -> Fcn/1
  Fcn/1 -> Product/1, Product1/1, Product2/1

== system Generator_Lib/VSCF Cycloconverter/AC Generator Cycloconverter/Ideal Source/Sensing ==
  Constant : Constant  Value=[1 1]*12000  SampleTime=-1
  Constant1 : Constant  Value=202  SampleTime=-1
  Mux : Mux  Inputs=3
  rpm2pu1 : Gain  Gain=2*pi/60
  tag scope: Gen1Data=global
  wires:
  [Pwr_Gen1_Only] -> Mux/3
  Constant1/1 -> Mux/2
  rpm2pu1/1 -> Mux/1
  Mux/1 -> [Gen1Data]
  Constant/1 -> rpm2pu1/1  "Spd"
